simulink model "pid_sim"  (R2020b)
settings: Solver=ode4  StartTime=0.0  StopTime=20  FixedStep=0.00001  RelTol=1e-3
values from neighbouring files (symbols this model uses):
  alpha = 1    [md.m]    (also in pid.m; pinolo.m)
  B = 0.05    [md.m]    (also in pid.m; pinolo.m)
  dt = 0.08    [md.m]    (also in pid.m; pinolo.m)
  J = 0.008    [md.m]    (also in pid.m; pinolo.m)
  kd = kd_sp(100,1)    [md.m]    (also in pid.m = 0.07; pinolo.m; pinolo_cmp.m = data{5})
  ki = ki_sp(100,1)    [md.m]    (also in pid.m = 7.15; pinolo.m; pinolo_cmp.m = data{4})
  KM = 0.22    [md.m]    (also in pid.m; pinolo.m)
  kp = kp_sp(100,1)    [md.m]    (also in pid.m = 1.43; pinolo.m; pinolo_cmp.m = data{3})
  L = 0.0014    [md.m]    (also in pid.m; pinolo.m)
  max_output = MAX_SPEED    (= 330)    [md.m]    (also in pid.m; pinolo.m)
  R = 2    [md.m]    (also in pid.m; pinolo.m)
undefined symbols (not defined in the file or in its folder): den, num
libraries: simulink x3
settings Model: NumberOfSteps=100000  Creator=Titania  LastModifiedBy=Titania

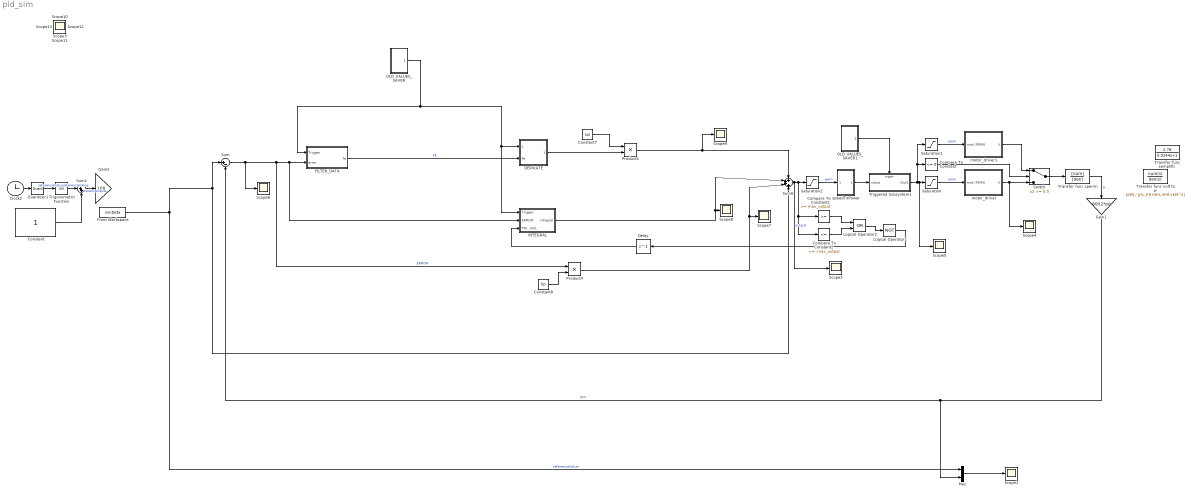
== system pid_sim ==
  Clock2 : Clock
  Compare To Constant : simulink/Logic and Bit Operations/Compare To Constant  relop=<=  const=0  OutDataTypeStr=boolean
  Compare To Constant1 : simulink/Logic and Bit Operations/Compare To Constant  relop=>=  const=max_output  OutDataTypeStr=boolean
  Compare To Constant2 : simulink/Logic and Bit Operations/Compare To Constant  relop=<=  const=-max_output  OutDataTypeStr=boolean
  Constant : Constant
  Constant7 : Constant  Value=kd
  Constant8 : Constant  Value=kp
  DERIVATE : Subsystem
  Delay : Delay  DelayLength=1  InitialCondition=0
  FILTER_DATA : Subsystem
  From Workspace : FromWorkspace  VariableName=simData
  Gain1 : Gain  Gain=60/(2*pi)
  Gain2 : Gain  Gain=100
  INTEGRAL : Subsystem
  Logical Operator1 : Logic  Operator=NOT  AllPortsSameDT=off  OutDataTypeStr=boolean
  Logical Operator2 : Logic  Operator=OR  AllPortsSameDT=off  OutDataTypeStr=boolean
  Mux : Mux  Inputs=2
  OLD_VALUES_SAVER : Subsystem
  OLD_VALUES_SAVER1 : Subsystem
  Product3 : Product  OutDataTypeStr=single
  Product4 : Product  OutDataTypeStr=single
  Quantizer1 : Quantizer  QuantizationInterval=1
  Saturation : Saturate  UpperLimit=1024  LowerLimit=0
  Saturation1 : Saturate  UpperLimit=0  LowerLimit=-1024
  Saturation2 : Saturate  UpperLimit=max_output  LowerLimit=-max_output
  Scope{,1..13} (14 alike) : Scope
  Sum : Sum  Inputs=|+-  OutDataTypeStr=single
  Sum1 : Sum  Inputs=|++
  Sum6 : Sum  Inputs=++++
  Switch : Switch  Threshold=0.5
  Transfer func semplific : TransferFcn  Numerator=2.78  Denominator=[0.0244,1]
  Transfer func sperim : TransferFcn  Numerator=[num]  Denominator=[den]
  Transfer func volt to w : TransferFcn  Numerator=[KM]  Denominator=[J*L,J*R+B*L,B*R+KM^2]
  Triggered Subsystem1 : Subsystem  TreatAsAtomicUnit=on
  Trigonometric Function : Trigonometry
  motor_driver : Subsystem
  motor_driver1 : Subsystem
  speedToPower : Subsystem
  wires:
  Sum/1 -> Scope6/1, Product4/1, INTEGRAL/2(ERROR), FILTER_DATA/2(error)  "ERROR"
  Product4/1 -> Scope7/1, Sum6/3
  Quantizer1/1 -> Trigonometric Function/1  "referenceValue"
  Constant8/1 -> Product4/2
  Clock2/1 -> Quantizer1/1
  Sum6/1 -> Compare To Constant2/1, Compare To Constant1/1, Saturation2/1, Scope2/1  "output"
  Gain1/1 -> Sum/2, Mux/2  "rpm"
  Mux/1 -> Scope1/1
  ? -> ?
  OLD_VALUES_SAVER/1(trigger) -> FILTER_DATA/1(Trigger), INTEGRAL/1(Trigger), DERIVATE/1(Trigger)
  Product3/1 -> Scope9/1, Sum6/1
  INTEGRAL/1(integral) -> Scope8/1, Sum6/2
  FILTER_DATA/1(fe) -> DERIVATE/2(fe)  "FE"
  Constant7/1 -> Product3/1
  DERIVATE/1(derivative) -> Product3/2
  motor_driver/1(V) -> Switch/3, Scope4/1
  Transfer func sperim/1 -> Gain1/1  "w"
  Triggered Subsystem1/1(Out1) -> Saturation1/1, Compare To Constant/1, Saturation/1, Scope5/1
  Saturation/1 -> motor_driver/1(mot (PWM))  "pwm"
  From Workspace/1 -> Sum6/4, Sum/1, Mux/1  "referenceValue"
  Trigonometric Function/1 -> Sum1/1  "referenceValue"
  Constant/1 -> Sum1/2
  Sum1/1 -> Gain2/1  "referenceValue"
  speedToPower/1(value) -> Triggered Subsystem1/1(value)
  OLD_VALUES_SAVER1/1(trigger) -> Triggered Subsystem1/Trigger
  Compare To Constant/1 -> Switch/2
  Switch/1 -> Transfer func sperim/1
  Saturation1/1 -> motor_driver1/1(mot (PWM))  "pwm"
  motor_driver1/1(V) -> Switch/1
  Saturation2/1 -> speedToPower/1(speed)  "pwm"
  Compare To Constant1/1 -> Logical Operator2/1
  Compare To Constant2/1 -> Logical Operator2/2
  Logical Operator2/1 -> Logical Operator1/1
  Logical Operator1/1 -> Delay/1
  Delay/1 -> INTEGRAL/3(TRIGGER_INTEGRAL)

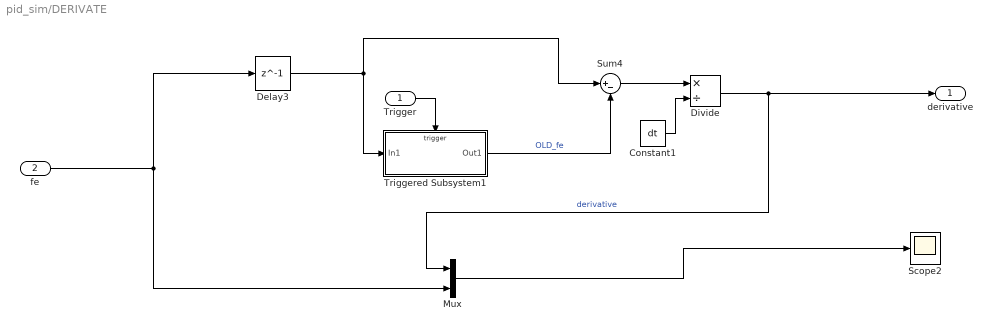
== system pid_sim/DERIVATE ==
  Trigger : Inport
  fe : Inport  Port=2
  Constant1 : Constant  Value=dt
  Delay3 : Delay  DelayLength=1  InitialCondition=0
  Divide : Product  Inputs=*/  OutDataTypeStr=single
  Mux : Mux  Inputs=2
  Scope2 : Scope
  Sum4 : Sum  Inputs=|+-
  Triggered Subsystem1 : Subsystem  TreatAsAtomicUnit=on
  derivative : Outport
  wires:
  fe/1 -> Mux/2, Delay3/1
  Sum4/1 -> Divide/1
  Delay3/1 -> Sum4/1, Triggered Subsystem1/1(In1)
  Triggered Subsystem1/1(Out1) -> Sum4/2  "OLD_fe"
  Trigger/1 -> Triggered Subsystem1/Trigger
  Constant1/1 -> Divide/2
  Divide/1 -> Mux/1, derivative/1  "derivative"
  Mux/1 -> Scope2/1

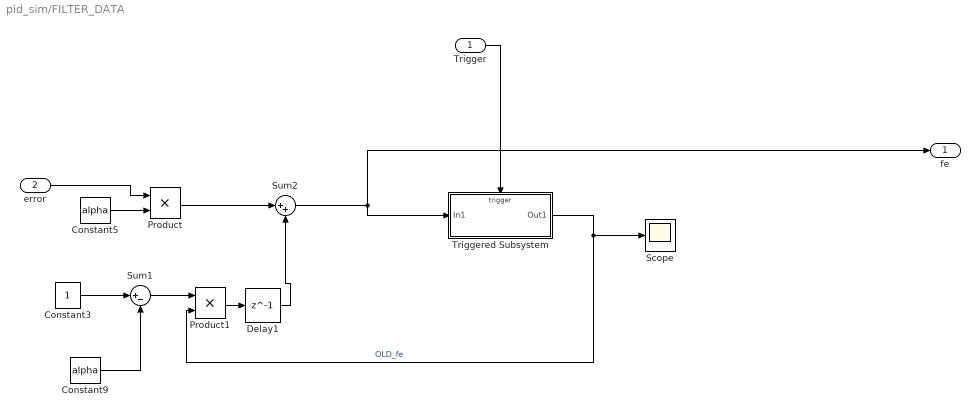
== system pid_sim/FILTER_DATA ==
  Trigger : Inport
  error : Inport  Port=2
  Constant3 : Constant
  Constant5 : Constant  Value=alpha
  Constant9 : Constant  Value=alpha
  Delay1 : Delay  DelayLength=1  InitialCondition=0
  Product : Product  OutDataTypeStr=single
  Product1 : Product  OutDataTypeStr=single
  Scope : Scope
  Sum1 : Sum  Inputs=|+-
  Sum2 : Sum  Inputs=|++
  Triggered Subsystem : Subsystem  TreatAsAtomicUnit=on
  fe : Outport
  wires:
  Sum2/1 -> fe/1, Triggered Subsystem/1(In1)
  Constant3/1 -> Sum1/1
  Product/1 -> Sum2/1
  Constant9/1 -> Sum1/2
  Triggered Subsystem/1(Out1) -> Product1/2, Scope/1  "OLD_fe"
  Sum1/1 -> Product1/1
  Trigger/1 -> Triggered Subsystem/Trigger
  Delay1/1 -> Sum2/2
  Constant5/1 -> Product/2
  Product1/1 -> Delay1/1
  error/1 -> Product/1

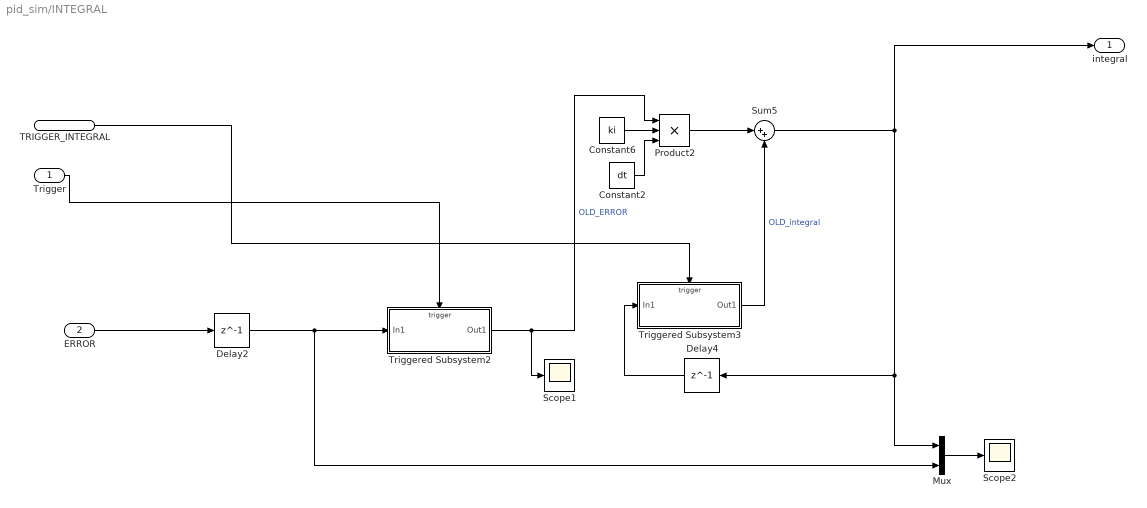
== system pid_sim/INTEGRAL ==
  Trigger : Inport
  ERROR : Inport  Port=2
  TRIGGER_INTEGRAL : Inport  Port=3
  Constant2 : Constant  Value=dt
  Constant6 : Constant  Value=ki
  Delay2 : Delay  DelayLength=1  InitialCondition=0
  Delay4 : Delay  DelayLength=1  InitialCondition=0
  Mux : Mux  Inputs=2
  Product2 : Product  Inputs=3  OutDataTypeStr=single
  Scope1 : Scope
  Scope2 : Scope
  Sum5 : Sum  Inputs=|++
  Triggered Subsystem2 : Subsystem  TreatAsAtomicUnit=on
  Triggered Subsystem3 : Subsystem  TreatAsAtomicUnit=on
  integral : Outport
  wires:
  Product2/1 -> Sum5/1
  Triggered Subsystem2/1(Out1) -> Scope1/1, Product2/1  "OLD_ERROR"
  Constant2/1 -> Product2/3
  Sum5/1 -> integral/1, Mux/1, Delay4/1
  Delay2/1 -> Mux/2, Triggered Subsystem2/1(In1)
  Delay4/1 -> Triggered Subsystem3/1(In1)
  Constant6/1 -> Product2/2
  Triggered Subsystem3/1(Out1) -> Sum5/2  "OLD_integral"
  Trigger/1 -> Triggered Subsystem2/Trigger
  ERROR/1 -> Delay2/1
  Mux/1 -> Scope2/1
  TRIGGER_INTEGRAL/1 -> Triggered Subsystem3/Trigger

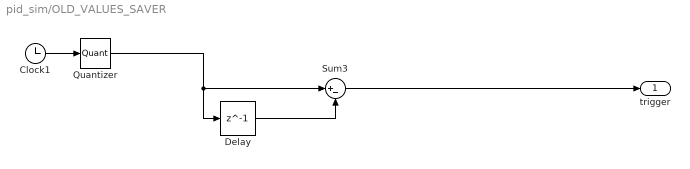
== system pid_sim/OLD_VALUES_SAVER ==
  Clock1 : Clock
  Delay : Delay  DelayLength=1  InitialCondition=0
  Quantizer : Quantizer  QuantizationInterval=dt
  Sum3 : Sum  Inputs=|+-  OutDataTypeStr=single
  trigger : Outport
  wires:
  Clock1/1 -> Quantizer/1
  Delay/1 -> Sum3/2
  Sum3/1 -> trigger/1
  Quantizer/1 -> Delay/1, Sum3/1

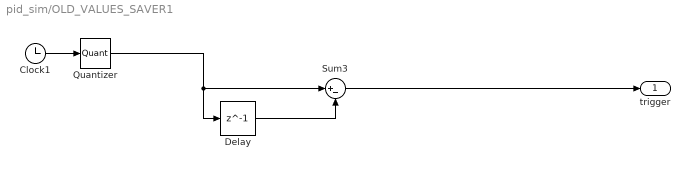
== system pid_sim/OLD_VALUES_SAVER1 ==
  Clock1 : Clock
  Delay : Delay  DelayLength=1  InitialCondition=0
  Quantizer : Quantizer  QuantizationInterval=dt_function
  Sum3 : Sum  Inputs=|+-  OutDataTypeStr=single
  trigger : Outport
  wires:
  Clock1/1 -> Quantizer/1
  Delay/1 -> Sum3/2
  Sum3/1 -> trigger/1
  Quantizer/1 -> Delay/1, Sum3/1

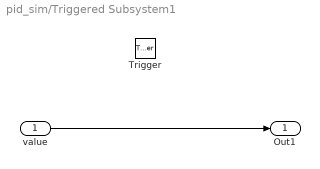
== system pid_sim/Triggered Subsystem1 ==
  value : Inport
  Trigger : TriggerPort  VariantControl=Variant
  Out1 : Outport
  wires:
  value/1 -> Out1/1

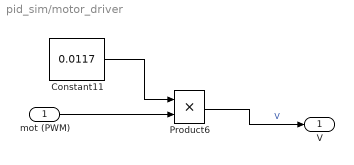
== system pid_sim/motor_driver ==
  mot (PWM) : Inport
  Constant11 : Constant  Value=0.0117
  Product6 : Product
  V : Outport
  wires:
  Constant11/1 -> Product6/1
  Product6/1 -> V/1  "V"
  mot (PWM)/1 -> Product6/2

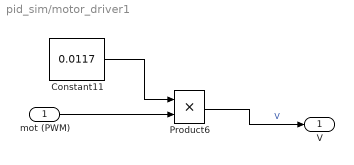
== system pid_sim/motor_driver1 ==
  mot (PWM) : Inport
  Constant11 : Constant  Value=0.0117
  Product6 : Product
  V : Outport
  wires:
  Constant11/1 -> Product6/1
  Product6/1 -> V/1  "V"
  mot (PWM)/1 -> Product6/2

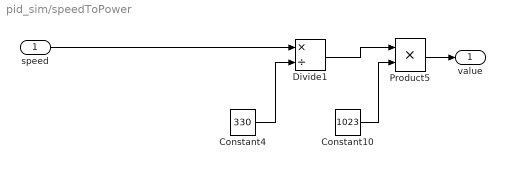
== system pid_sim/speedToPower ==
  speed : Inport
  Constant10 : Constant  Value=1023
  Constant4 : Constant  Value=330
  Divide1 : Product  Inputs=*/  OutDataTypeStr=single
  Product5 : Product  OutDataTypeStr=single
  value : Outport
  wires:
  speed/1 -> Divide1/1
  Divide1/1 -> Product5/1
  Product5/1 -> value/1
  Constant10/1 -> Product5/2
  Constant4/1 -> Divide1/2

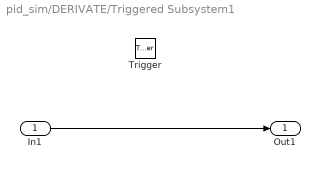
== system pid_sim/DERIVATE/Triggered Subsystem1 ==
  In1 : Inport
  Trigger : TriggerPort  VariantControl=Variant
  Out1 : Outport
  wires:
  In1/1 -> Out1/1

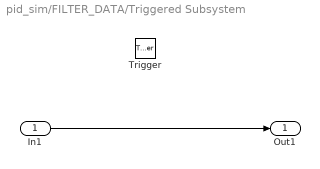
== system pid_sim/FILTER_DATA/Triggered Subsystem ==
  In1 : Inport
  Trigger : TriggerPort  VariantControl=Variant
  Out1 : Outport
  wires:
  In1/1 -> Out1/1

== system pid_sim/INTEGRAL/Triggered Subsystem2 ==
  In1 : Inport
  Trigger : TriggerPort  VariantControl=Variant
  Out1 : Outport
  wires:
  In1/1 -> Out1/1

== system pid_sim/INTEGRAL/Triggered Subsystem3 ==
  In1 : Inport
  Trigger : TriggerPort  VariantControl=Variant
  Out1 : Outport
  wires:
  In1/1 -> Out1/1
